simulink model "fuzzy_pid"  (Simulink 6.4)
settings: Solver=ode45  StartTime=0.0  StopTime=10.0  RelTol=1e-3
libraries: fuzblock x1
settings Model: LastModifiedBy=Administrator

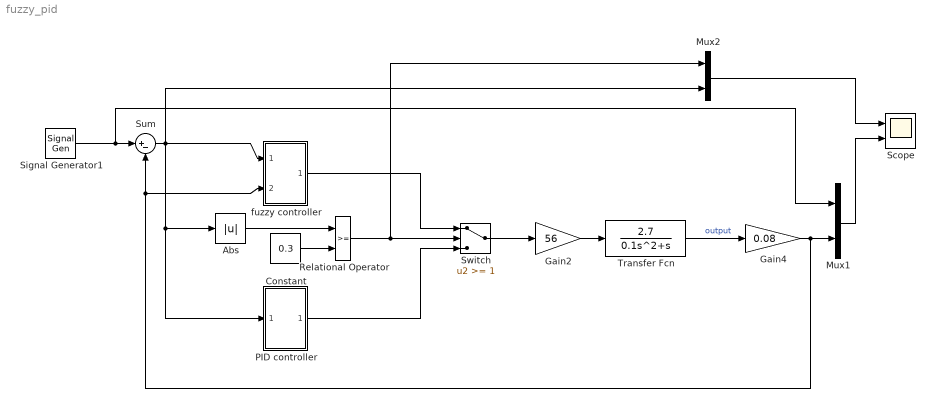
== system fuzzy_pid ==
  Abs : Abs  SaturateOnIntegerOverflow=on  SampleTime=-1
  Constant : Constant  Value=0.3  OutDataType=sfix(16)  ConRadixGroup=Use specified scaling  OutScaling=2^0  SampleTime=inf  FramePeriod=inf
  Gain2 : Gain  Gain=56  SaturateOnIntegerOverflow=on
  Gain4 : Gain  Gain=0.08  SaturateOnIntegerOverflow=on
  Mux1 : Mux  Inputs=2
  Mux2 : Mux  Inputs=2
  "PID controller " : Subsystem
  Relational Operator : RelationalOperator  InputSameDT=on
  Scope : Scope  NumInputPorts=2
      settings: TimeRange=0.1  YMin=0.935~5.55112e-017  YMax=1~1  MaxDataPoints=30000
  Signal Generator1 : SignalGenerator  Units=rad/sec
  Sum : Sum  Inputs=|+-  SaturateOnIntegerOverflow=on  InputSameDT=on
  Switch : Switch  Threshold=1  SaturateOnIntegerOverflow=on  InputSameDT=on
  Transfer Fcn : TransferFcn  Numerator=[2.7]  Denominator=[0.1 1 0]
  fuzzy controller : Subsystem
  wires:
  Transfer Fcn/1 -> Gain4/1  "output"
  Mux1/1 -> Scope/2
  Gain2/1 -> Transfer Fcn/1
  Gain4/1 -> Mux1/2, Sum/2, fuzzy controller/2(In2)
  Sum/1 -> fuzzy controller/1(In1), "PID controller "/1(In1), Abs/1, Mux2/2
  Signal Generator1/1 -> Sum/1, Mux1/1
  fuzzy controller/1(Out1) -> Switch/1
  "PID controller "/1(Out1) -> Switch/3
  Switch/1 -> Gain2/1
  Constant/1 -> Relational Operator/2
  Relational Operator/1 -> Switch/2, Mux2/1
  Mux2/1 -> Scope/1
  Abs/1 -> Relational Operator/1

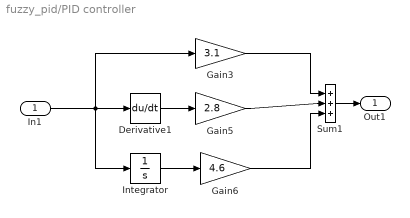
== system fuzzy_pid/PID controller  ==
  In1 : Inport
  Derivative1 : Derivative
  Gain3 : Gain  Gain=3.1  SaturateOnIntegerOverflow=on
  Gain5 : Gain  Gain=2.8  SaturateOnIntegerOverflow=on
  Gain6 : Gain  Gain=4.6  SaturateOnIntegerOverflow=on
  Integrator : Integrator
  Sum1 : Sum  Inputs=|+++  SaturateOnIntegerOverflow=on  InputSameDT=on
  Out1 : Outport
  wires:
  Derivative1/1 -> Gain5/1
  Integrator/1 -> Gain6/1
  Gain3/1 -> Sum1/1
  Gain5/1 -> Sum1/2
  Gain6/1 -> Sum1/3
  Sum1/1 -> Out1/1
  In1/1 -> Gain3/1, Integrator/1, Derivative1/1

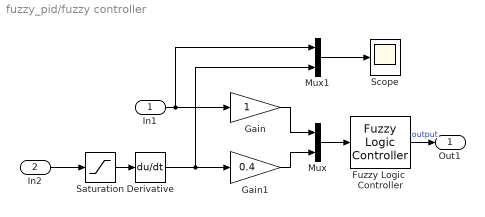
== system fuzzy_pid/fuzzy controller ==
  In1 : Inport
  In2 : Inport  Port=2
  Derivative : Derivative
  Fuzzy Logic  Controller : fuzblock/Fuzzy Logic  Controller  SystemSampleTime=-1  fis=demo1
  Gain : Gain  SaturateOnIntegerOverflow=on
  Gain1 : Gain  Gain=0.4  SaturateOnIntegerOverflow=on
  Mux : Mux  Inputs=2
  Mux1 : Mux  Inputs=2
  Saturation : Saturate  UpperLimit=10  LowerLimit=-10
  Scope : Scope
      settings: TimeRange=1  YMin=0  YMax=2.5  MaxDataPoints=30000
  Out1 : Outport
  wires:
  Derivative/1 -> Gain1/1, Mux1/2
  Gain/1 -> Mux/1
  Mux/1 -> Fuzzy Logic  Controller/1
  Gain1/1 -> Mux/2
  Saturation/1 -> Derivative/1
  In1/1 -> Gain/1, Mux1/1
  In2/1 -> Saturation/1
  Fuzzy Logic  Controller/1 -> Out1/1  "output"
  Mux1/1 -> Scope/1
